simulink model "position"  (R2024a)
settings: Solver=VariableStepAuto  StartTime=0.0  StopTime=3  RelTol=1e-3
settings Model: Creator=George  LastModifiedBy=volko
settings RTWCC: GPUComputeCapability=3.5

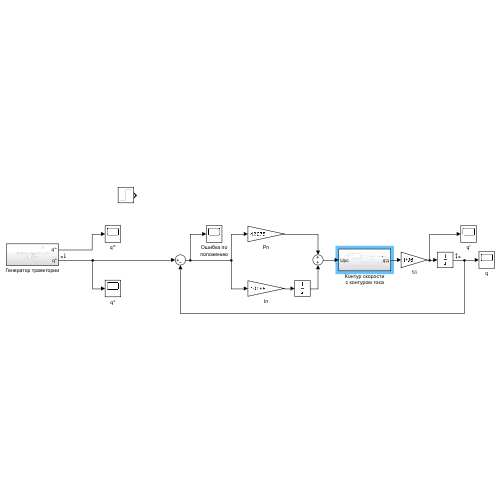
[thumbnail: Simulink's stored preview of the top-level diagram]
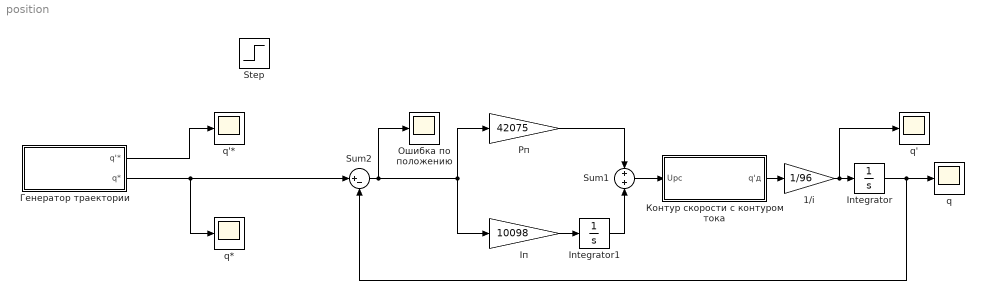
== system position ==
  1/i : Gain  Gain=1/96
  Integrator : Integrator
  Integrator1 : Integrator
  Iп : Gain  Gain=10098
  Pп : Gain  Gain=42075
  Step : Step  Time=0.05  SampleTime=0
  Sum1 : Sum
  Sum2 : Sum  Inputs=|+-
  q : Scope
  q' : Scope
  q'* : Scope
  q* : Scope
  Генератор траектории : Subsystem
  Контур скорости с контуром тока : Subsystem
  Ошибка по положению : Scope
  wires:
  Контур скорости с контуром тока/1(q'д) -> 1/i/1
  1/i/1 -> q'/1, Integrator/1
  Iп/1 -> Integrator1/1
  Integrator/1 -> Sum2/2, q/1
  Sum2/1 -> Ошибка по положению/1, Pп/1, Iп/1
  Sum1/1 -> Контур скорости с контуром тока/1(Uрс)
  Pп/1 -> Sum1/1
  Генератор траектории/1(q'*) -> q'*/1
  Integrator1/1 -> Sum1/2
  Генератор траектории/2(q*) -> q*/1, Sum2/1

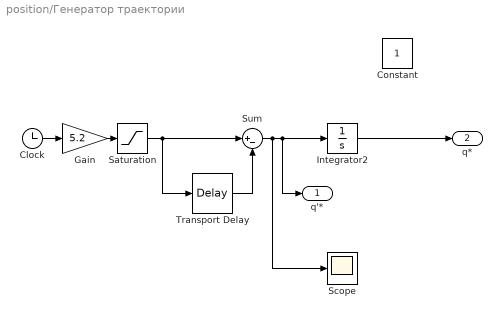
== system position/Генератор траектории ==
  Clock : Clock
  Constant : Constant
  Gain : Gain  Gain=5.2
  Integrator2 : Integrator
  Saturation : Saturate  UpperLimit=700  LowerLimit=0
  Scope : Scope
  Sum : Sum  Inputs=|+-
  Transport Delay : TransportDelay  DelayTime=1.5
  q'* : Outport
  q* : Outport  Port=2
  wires:
  Clock/1 -> Gain/1
  Gain/1 -> Saturation/1
  Saturation/1 -> Sum/1, Transport Delay/1
  Transport Delay/1 -> Sum/2
  Sum/1 -> Scope/1, Integrator2/1, q'*/1
  Integrator2/1 -> q*/1

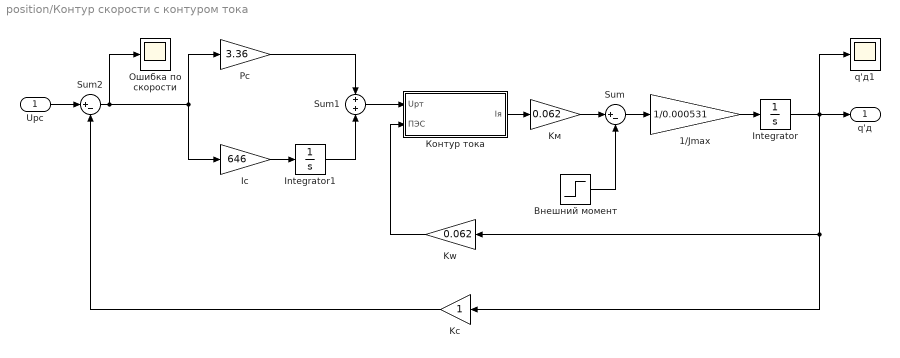
== system position/Контур скорости с контуром тока ==
  Uрс : Inport
  1/Jmax : Gain  Gain=1/0.000531
  Integrator : Integrator
  Integrator1 : Integrator
  Iс : Gain  Gain=646
  Kw : Gain  Gain=0.062
  Kм : Gain  Gain=0.062
  Kс : Gain
  Pс : Gain  Gain=3.36
  Sum : Sum  Inputs=|+-
  Sum1 : Sum
  Sum2 : Sum  Inputs=|+-
  q'д1 : Scope
  Внешний момент : Step  After=0.47  SampleTime=0
  Контур тока : Subsystem
  Ошибка по скорости : Scope
  q'д : Outport
  wires:
  Uрс/1 -> Sum2/1
  Pс/1 -> Sum1/1
  Sum1/1 -> Контур тока/1(Uрт)
  1/Jmax/1 -> Integrator/1
  Integrator/1 -> q'д1/1, q'д/1, Kс/1, Kw/1
  Integrator1/1 -> Sum1/2
  Внешний момент/1 -> Sum/2
  Sum2/1 -> Ошибка по скорости/1, Pс/1, Iс/1
  Контур тока/1(Iя) -> Kм/1
  Kм/1 -> Sum/1
  Kс/1 -> Sum2/2
  Sum/1 -> 1/Jmax/1
  Iс/1 -> Integrator1/1
  Kw/1 -> Контур тока/2(ПЭС)

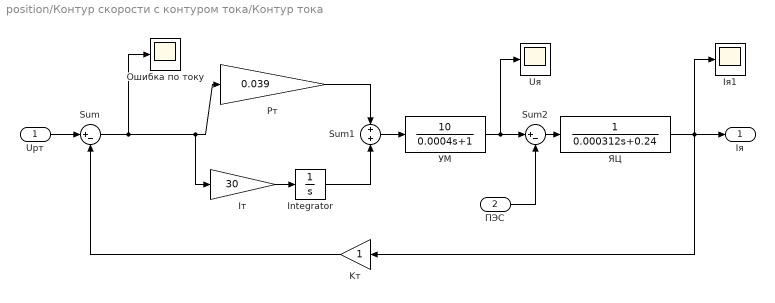
== system position/Контур скорости с контуром тока/Контур тока ==
  Uрт : Inport
  ПЭС : Inport  Port=2
  Integrator : Integrator
  Iт : Gain  Gain=30
  Iя1 : Scope
  Kт : Gain
  Pт : Gain  Gain=0.039
  Sum : Sum  Inputs=|+-
  Sum1 : Sum
  Sum2 : Sum  Inputs=|+-
  Uя : Scope
  Ошибка по току : Scope
  УМ : TransferFcn  Numerator=[10]  Denominator=[0.0004 1]
  ЯЦ : TransferFcn  Denominator=[0.000312 0.24]
  Iя : Outport
  wires:
  УМ/1 -> Sum2/1, Uя/1
  Integrator/1 -> Sum1/2
  Sum1/1 -> УМ/1
  Iт/1 -> Integrator/1
  Sum/1 -> Ошибка по току/1, Iт/1, Pт/1
  ЯЦ/1 -> Iя1/1, Iя/1, Kт/1
  Kт/1 -> Sum/2
  Pт/1 -> Sum1/1
  Uрт/1 -> Sum/1
  Sum2/1 -> ЯЦ/1
  ПЭС/1 -> Sum2/2
